simulink model "ctrl_HSMBObserver"  (R2015a)
settings: Solver=ode3  StartTime=0.0  StopTime=inf  FixedStep=0.01  RelTol=1e-3
values from neighbouring files (symbols this model uses):
  C = [C1;C2;C3;C4;C5;C6]    [initfile.m]    (also in thrustallocationQuadraticFixed.m)
  D = 3.0/100    (= 0.03)    [initfile.m]    (also in thrustallocationQuadraticFixed.m = 0.0411111111111)
  eps_c = 5    [initfile.m]
  epsilon = 0.5    [initfile.m]    (also in thrustallocationPseudo.m = u(10); thrustallocationQuadraticFixed.m = u(10))
  hd = c2d(H1,0.01,'foh')    [initfile.m]
  hd2 = c2d(H2,0.01,'zoh')    [initfile.m]
  I_s = 25000 /747225    (= 0.0334571246947)    [initfile.m]
  k_cc = 1    [initfile.m]
  K_omega = 0.3    [initfile.m]
  K_q1f = 0.0113    [initfile.m]
  K_q1r = K_q1f    (= 0.0113)    [initfile.m]
  K_q2f = 0.0117    [initfile.m]
  K_q2r = K_q2f    (= 0.0117)    [initfile.m]
  K_q3f = 0.0113    [initfile.m]
  K_q3r = K_q3f    (= 0.0113)    [initfile.m]
  K_q4f = 0.0169    [initfile.m]
  K_q4r = K_q4f    (= 0.0169)    [initfile.m]
  K_q5f = 0.0144    [initfile.m]
  K_q5r = K_q5f    (= 0.0144)    [initfile.m]
  K_q6f = 0.0168    [initfile.m]
  K_q6r = K_q6f    (= 0.0168)    [initfile.m]
  K_T1f = 0.3763    [initfile.m]
  K_T1r = K_T1f    (= 0.3763)    [initfile.m]
  K_T2f = 0.3901    [initfile.m]
  K_T2r = K_T2f    (= 0.3901)    [initfile.m]
  K_T3f = 0.3776    [initfile.m]
  K_T3r = K_T3f    (= 0.3776)    [initfile.m]
  K_T4f = 0.5641    [initfile.m]
  K_T4r = K_T4f    (= 0.5641)    [initfile.m]
  K_T5f = 0.4799    [initfile.m]
  K_T5r = K_T5f    (= 0.4799)    [initfile.m]
  K_T6f = 0.5588    [initfile.m]
  K_T6r = K_T6f    (= 0.5588)    [initfile.m]
  Kp = 3.3    [initfile.m]
  Max_Acceleration = 5    [initfile.m]
  Max_rotation = 12*sqrt(lambda)    [initfile.m]
  Max_thrust = 1.5    [initfile.m]
  Min_thrust = -0.8    [initfile.m]
  n_c = 5    [initfile.m]
  n_max = 152    [initfile.m]
  p_cc = 0.5    [initfile.m]
  pwm_thr1_backward = coeffvalues(ForceToPWM)    [initfile.m]
  pwm_thr1_forward = coeffvalues(ForceToPWM)    [initfile.m]
  pwm_thr2_backward = coeffvalues(ForceToPWM)    [initfile.m]
  pwm_thr2_forward = coeffvalues(ForceToPWM)    [initfile.m]
  pwm_thr3_backward = coeffvalues(ForceToPWM)    [initfile.m]
  pwm_thr3_forward = coeffvalues(ForceToPWM)    [initfile.m]
  pwm_thr4_backward = coeffvalues(ForceToPWM)    [initfile.m]
  pwm_thr4_forward = coeffvalues(ForceToPWM)    [initfile.m]
  pwm_thr5_backward = coeffvalues(ForceToPWM)    [initfile.m]
  pwm_thr5_forward = coeffvalues(ForceToPWM)    [initfile.m]
  pwm_thr6_backward = coeffvalues(ForceToPWM)    [initfile.m]
  pwm_thr6_forward = coeffvalues(ForceToPWM)    [initfile.m]
  Q_f0 = 0.3    [initfile.m]
  r_cc = 4    [initfile.m]
  Rho = Rho_m    (= 1000)    [initfile.m]
  ts = [-1 0]    [thrustallocationPseudo.m]    (also in thrustallocationQuadraticFixed.m)
undefined symbols (not defined in the file or in its folder): AFB, arm, Att, Control, Damping, FaultDet, Glob, Grip, IntActionType, Mass, NPO, Obs, Omg0_min, Q_max, ReferenceMdl, Sensor, Sim, SwLogic, tau, Thruster, Thruster_lock
libraries: dspmtrx3 x14, marine_gnc x11, simulink_extras x9, dspstat3 x9, simulink x9, dsparch4 x6, dspspect3 x6
(part 4 of 7)

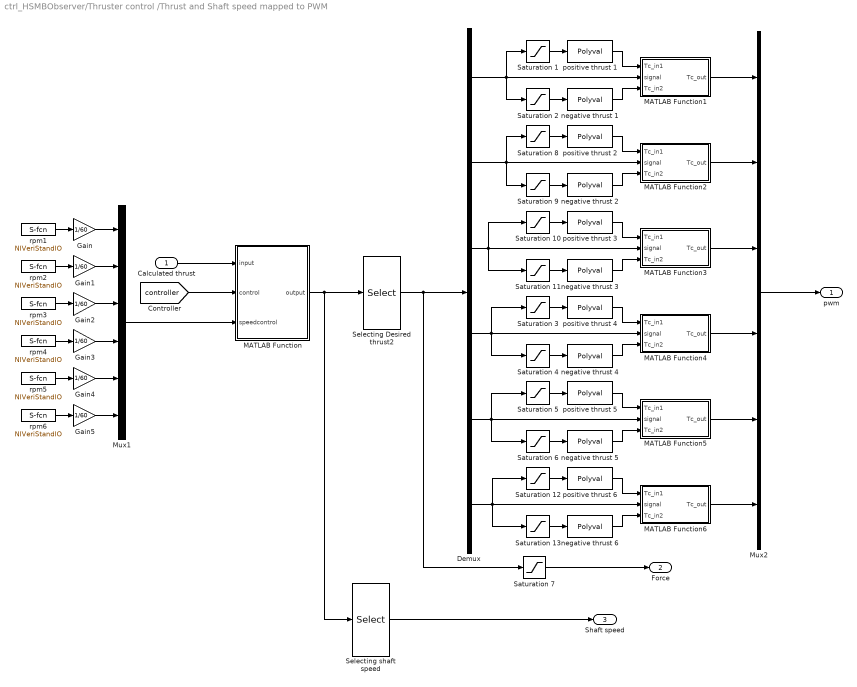
== system ctrl_HSMBObserver/Thruster control /Thrust and Shaft speed mapped to PWM ==
  Calculated thrust : Inport
  Demux : Demux  Outputs=6
  Gain{,1..5} (6 alike) : Gain  Gain=1/60
  MATLAB Function : MATLAB Function  TreatAsAtomicUnit=on
  MATLAB Function1 : MATLAB Function  TreatAsAtomicUnit=on
  MATLAB Function2 : MATLAB Function  TreatAsAtomicUnit=on
  MATLAB Function3 : MATLAB Function  TreatAsAtomicUnit=on
  MATLAB Function4 : MATLAB Function  TreatAsAtomicUnit=on
  MATLAB Function5 : MATLAB Function  TreatAsAtomicUnit=on
  MATLAB Function6 : MATLAB Function  TreatAsAtomicUnit=on
  Mux1 : Mux  Inputs=6
  Mux2 : Mux  Inputs=6
  Saturation {1,3,5,8,10,12} (6 alike) : Saturate  UpperLimit=Max_thrust  LowerLimit=0
  Saturation {2,4,6,9,11,13} (6 alike) : Saturate  UpperLimit=0  LowerLimit=Min_thrust
  Saturation 7 : Saturate  UpperLimit=Max_thrust  LowerLimit=-Max_thrust
  Selecting Desired thrust2 : Selector  InputPortWidth=12  Indices=[1 3 5 7 9 11]
  Selecting shaft speed : Selector  InputPortWidth=12  Indices=[2 4 6 8 10 12]
  negative thrust 1 : Polyval  Coefs=pwm_thr1_backward
  negative thrust 2 : Polyval  Coefs=pwm_thr2_backward
  negative thrust 3 : Polyval  Coefs=pwm_thr3_backward
  negative thrust 4 : Polyval  Coefs=pwm_thr4_backward
  negative thrust 5 : Polyval  Coefs=pwm_thr5_backward
  negative thrust 6 : Polyval  Coefs=pwm_thr6_backward
  positive thrust 1 : Polyval  Coefs=pwm_thr1_forward
  positive thrust 2 : Polyval  Coefs=pwm_thr2_forward
  positive thrust 3 : Polyval  Coefs=pwm_thr3_forward
  positive thrust 4 : Polyval  Coefs=pwm_thr4_forward
  positive thrust 5 : Polyval  Coefs=pwm_thr5_forward
  positive thrust 6 : Polyval  Coefs=pwm_thr6_forward
  "rpm1 " : S-Function  Priority=1  FunctionName=NIVeriStandIO  Parameters=width dtype portnum stime stype btype  mask(NI VeriStand Inport){portnum=1, width=-1, stime=-1, dtype=auto, stype=auto, btype=1}
      mask prompts: portnum "Port number:"; width "Port dimensions (-1 for dynamically sized):"; stime "Sample time (-1 for inherited):"; dtype "Data type:"; stype "Signal type:"; btype "Block type:"
      mask help: Use this inport on any level of nested subsystems to allow NI VeriStand software to map signals to it.
      mask init:
      | NIVeriStandIO_init;
      settings: CopyFcn=NIVeriStand_MDL_functions('', 'IO_copy');  DeleteFcn=NIVeriStand_MDL_functions('', 'IO_delete');  MoveFcn=set_param(gcb, 'Mask', 'on');
      mask Callback portnum: NIVeriStand_MDL_functions('', 'IO_setportnum');
      mask TypeOptions dtype: auto | double | single | int8 | uint8 | int16 | uint16 | int32 | uint32 | boolean
      mask Callback dtype: NIVeriStand_MDL_functions('', 'IO_booleansignal');
      mask TypeOptions stype: auto | real | complex
      mask Display:
      | patch([-x x], [-y y], [.90980 .81960 .32156]);
      | plot([xrad -x x xrad], [yrad -y y yrad]);
      | fprintf('NI In%d', portnum);
  rpm2 : S-Function  Priority=2  FunctionName=NIVeriStandIO  Parameters=width dtype portnum stime stype btype  mask(NI VeriStand Inport){portnum=2, width=-1, stime=-1, dtype=auto, stype=auto, btype=1}
      mask prompts: portnum "Port number:"; width "Port dimensions (-1 for dynamically sized):"; stime "Sample time (-1 for inherited):"; dtype "Data type:"; stype "Signal type:"; btype "Block type:"
      mask help: Use this inport on any level of nested subsystems to allow NI VeriStand software to map signals to it.
      mask init:
      | NIVeriStandIO_init;
      settings: CopyFcn=NIVeriStand_MDL_functions('', 'IO_copy');  DeleteFcn=NIVeriStand_MDL_functions('', 'IO_delete');  MoveFcn=set_param(gcb, 'Mask', 'on');
      mask Callback portnum: NIVeriStand_MDL_functions('', 'IO_setportnum');
      mask TypeOptions dtype: auto | double | single | int8 | uint8 | int16 | uint16 | int32 | uint32 | boolean
      mask Callback dtype: NIVeriStand_MDL_functions('', 'IO_booleansignal');
      mask TypeOptions stype: auto | real | complex
      mask Display:
      | patch([-x x], [-y y], [.90980 .81960 .32156]);
      | plot([xrad -x x xrad], [yrad -y y yrad]);
      | fprintf('NI In%d', portnum);
  rpm3 : S-Function  Priority=3  FunctionName=NIVeriStandIO  Parameters=width dtype portnum stime stype btype  mask(NI VeriStand Inport){portnum=3, width=-1, stime=-1, dtype=auto, stype=auto, btype=1}
      mask prompts: portnum "Port number:"; width "Port dimensions (-1 for dynamically sized):"; stime "Sample time (-1 for inherited):"; dtype "Data type:"; stype "Signal type:"; btype "Block type:"
      mask help: Use this inport on any level of nested subsystems to allow NI VeriStand software to map signals to it.
      mask init:
      | NIVeriStandIO_init;
      settings: CopyFcn=NIVeriStand_MDL_functions('', 'IO_copy');  DeleteFcn=NIVeriStand_MDL_functions('', 'IO_delete');  MoveFcn=set_param(gcb, 'Mask', 'on');
      mask Callback portnum: NIVeriStand_MDL_functions('', 'IO_setportnum');
      mask TypeOptions dtype: auto | double | single | int8 | uint8 | int16 | uint16 | int32 | uint32 | boolean
      mask Callback dtype: NIVeriStand_MDL_functions('', 'IO_booleansignal');
      mask TypeOptions stype: auto | real | complex
      mask Display:
      | patch([-x x], [-y y], [.90980 .81960 .32156]);
      | plot([xrad -x x xrad], [yrad -y y yrad]);
      | fprintf('NI In%d', portnum);
  rpm4 : S-Function  Priority=4  FunctionName=NIVeriStandIO  Parameters=width dtype portnum stime stype btype  mask(NI VeriStand Inport){portnum=4, width=-1, stime=-1, dtype=auto, stype=auto, btype=1}
      mask prompts: portnum "Port number:"; width "Port dimensions (-1 for dynamically sized):"; stime "Sample time (-1 for inherited):"; dtype "Data type:"; stype "Signal type:"; btype "Block type:"
      mask help: Use this inport on any level of nested subsystems to allow NI VeriStand software to map signals to it.
      mask init:
      | NIVeriStandIO_init;
      settings: CopyFcn=NIVeriStand_MDL_functions('', 'IO_copy');  DeleteFcn=NIVeriStand_MDL_functions('', 'IO_delete');  MoveFcn=set_param(gcb, 'Mask', 'on');
      mask Callback portnum: NIVeriStand_MDL_functions('', 'IO_setportnum');
      mask TypeOptions dtype: auto | double | single | int8 | uint8 | int16 | uint16 | int32 | uint32 | boolean
      mask Callback dtype: NIVeriStand_MDL_functions('', 'IO_booleansignal');
      mask TypeOptions stype: auto | real | complex
      mask Display:
      | patch([-x x], [-y y], [.90980 .81960 .32156]);
      | plot([xrad -x x xrad], [yrad -y y yrad]);
      | fprintf('NI In%d', portnum);
  rpm5 : S-Function  Priority=5  FunctionName=NIVeriStandIO  Parameters=width dtype portnum stime stype btype  mask(NI VeriStand Inport){portnum=5, width=-1, stime=-1, dtype=auto, stype=auto, btype=1}
      mask prompts: portnum "Port number:"; width "Port dimensions (-1 for dynamically sized):"; stime "Sample time (-1 for inherited):"; dtype "Data type:"; stype "Signal type:"; btype "Block type:"
      mask help: Use this inport on any level of nested subsystems to allow NI VeriStand software to map signals to it.
      mask init:
      | NIVeriStandIO_init;
      settings: CopyFcn=NIVeriStand_MDL_functions('', 'IO_copy');  DeleteFcn=NIVeriStand_MDL_functions('', 'IO_delete');  MoveFcn=set_param(gcb, 'Mask', 'on');
      mask Callback portnum: NIVeriStand_MDL_functions('', 'IO_setportnum');
      mask TypeOptions dtype: auto | double | single | int8 | uint8 | int16 | uint16 | int32 | uint32 | boolean
      mask Callback dtype: NIVeriStand_MDL_functions('', 'IO_booleansignal');
      mask TypeOptions stype: auto | real | complex
      mask Display:
      | patch([-x x], [-y y], [.90980 .81960 .32156]);
      | plot([xrad -x x xrad], [yrad -y y yrad]);
      | fprintf('NI In%d', portnum);
  rpm6 : S-Function  Priority=6  FunctionName=NIVeriStandIO  Parameters=width dtype portnum stime stype btype  mask(NI VeriStand Inport){portnum=6, width=-1, stime=-1, dtype=auto, stype=auto, btype=1}
      mask prompts: portnum "Port number:"; width "Port dimensions (-1 for dynamically sized):"; stime "Sample time (-1 for inherited):"; dtype "Data type:"; stype "Signal type:"; btype "Block type:"
      mask help: Use this inport on any level of nested subsystems to allow NI VeriStand software to map signals to it.
      mask init:
      | NIVeriStandIO_init;
      settings: CopyFcn=NIVeriStand_MDL_functions('', 'IO_copy');  DeleteFcn=NIVeriStand_MDL_functions('', 'IO_delete');  MoveFcn=set_param(gcb, 'Mask', 'on');
      mask Callback portnum: NIVeriStand_MDL_functions('', 'IO_setportnum');
      mask TypeOptions dtype: auto | double | single | int8 | uint8 | int16 | uint16 | int32 | uint32 | boolean
      mask Callback dtype: NIVeriStand_MDL_functions('', 'IO_booleansignal');
      mask TypeOptions stype: auto | real | complex
      mask Display:
      | patch([-x x], [-y y], [.90980 .81960 .32156]);
      | plot([xrad -x x xrad], [yrad -y y yrad]);
      | fprintf('NI In%d', portnum);
  pwm : Outport
  Force : Outport  Port=2
  "Shaft speed " : Outport  Port=3
  wires:
  MATLAB Function/1(output) -> Selecting shaft speed/1, Selecting Desired thrust2/1
  [controller] -> MATLAB Function/2(control)
  Mux2/1 -> pwm/1
  Selecting Desired thrust2/1 -> Saturation 7/1, Demux/1
  Selecting shaft speed/1 -> "Shaft speed "/1
  Saturation 7/1 -> Force/1
  "rpm1 "/1 -> Gain/1
  rpm2/1 -> Gain1/1
  rpm3/1 -> Gain2/1
  rpm4/1 -> Gain3/1
  rpm5/1 -> Gain4/1
  rpm6/1 -> Gain5/1
  Mux1/1 -> MATLAB Function/3(speedcontrol)
  positive thrust 1/1 -> MATLAB Function1/1(Tc_in1)
  negative thrust 1/1 -> MATLAB Function1/3(Tc_in2)
  Demux/1 -> Saturation 1/1, MATLAB Function1/2(signal), Saturation 2/1
  MATLAB Function1/1(Tc_out) -> Mux2/1
  Saturation 1/1 -> positive thrust 1/1
  Saturation 2/1 -> negative thrust 1/1
  positive thrust 2/1 -> MATLAB Function2/1(Tc_in1)
  negative thrust 2/1 -> MATLAB Function2/3(Tc_in2)
  Demux/2 -> Saturation 9/1, Saturation 8/1, MATLAB Function2/2(signal)
  MATLAB Function2/1(Tc_out) -> Mux2/2
  Saturation 8/1 -> positive thrust 2/1
  Saturation 9/1 -> negative thrust 2/1
  positive thrust 3/1 -> MATLAB Function3/1(Tc_in1)
  negative thrust 3/1 -> MATLAB Function3/3(Tc_in2)
  Demux/3 -> Saturation 11/1, MATLAB Function3/2(signal), Saturation 10/1
  MATLAB Function3/1(Tc_out) -> Mux2/3
  Saturation 10/1 -> positive thrust 3/1
  Saturation 11/1 -> negative thrust 3/1
  positive thrust 4/1 -> MATLAB Function4/1(Tc_in1)
  negative thrust 4/1 -> MATLAB Function4/3(Tc_in2)
  MATLAB Function4/1(Tc_out) -> Mux2/4
  Saturation 3/1 -> positive thrust 4/1
  Saturation 4/1 -> negative thrust 4/1
  Demux/4 -> Saturation 3/1, Saturation 4/1, MATLAB Function4/2(signal)
  positive thrust 5/1 -> MATLAB Function5/1(Tc_in1)
  negative thrust 5/1 -> MATLAB Function5/3(Tc_in2)
  MATLAB Function5/1(Tc_out) -> Mux2/5
  Saturation 5/1 -> positive thrust 5/1
  Saturation 6/1 -> negative thrust 5/1
  Demux/5 -> Saturation 5/1, MATLAB Function5/2(signal), Saturation 6/1
  positive thrust 6/1 -> MATLAB Function6/1(Tc_in1)
  negative thrust 6/1 -> MATLAB Function6/3(Tc_in2)
  MATLAB Function6/1(Tc_out) -> Mux2/6
  Saturation 12/1 -> positive thrust 6/1
  Saturation 13/1 -> negative thrust 6/1
  Demux/6 -> Saturation 13/1, Saturation 12/1, MATLAB Function6/2(signal)
  Gain/1 -> Mux1/1
  Gain5/1 -> Mux1/6
  Gain4/1 -> Mux1/5
  Gain3/1 -> Mux1/4
  Gain2/1 -> Mux1/3
  Gain1/1 -> Mux1/2
  Calculated thrust/1 -> MATLAB Function/1(input)

== system ctrl_HSMBObserver/Thruster control /Thruster 1 ==
  Desired thrust 1 : Inport
  shaft speed : Inport  Port=2
  Constant : Constant  Value=hd2.den{1,1}
  Constant1 : Constant  Value=hd2.num{1,1}
  Delay : Delay  DelayLength=1  InitialCondition=0
  Discrete Transfer Fcn : DiscreteTransferFcn  NumeratorSource=Input port  DenominatorSource=Input port  Denominator=[0.2 1]  SampleTime=0.01  a0EqualsOne=on
      settings: InputPortMap=u0,p1,p3
  Losses (placeholder) : Constant  Value=0
  Propeller Hydrodynamics : Subsystem
  Shaft dynamics : Subsystem
  Thruster control : Subsystem
  "Commanded thrust " : Outport
  Shaft speed : Outport  Port=2
  wires:
  Losses (placeholder)/1 -> Propeller Hydrodynamics/1(env)
  Shaft dynamics/1(n) -> Shaft speed/1, Propeller Hydrodynamics/2(n)
  Propeller Hydrodynamics/2(Qa) -> Delay/1
  Propeller Hydrodynamics/1(Ta) -> "Commanded thrust "/1
  Thruster control/1(Qc) -> Discrete Transfer Fcn/1
  Constant1/1 -> Discrete Transfer Fcn/2
  Constant/1 -> Discrete Transfer Fcn/3
  Discrete Transfer Fcn/1 -> Shaft dynamics/1(Qm)
  shaft speed/1 -> Thruster control/2(n)
  Delay/1 -> Shaft dynamics/2(Qa)
  Desired thrust 1/1 -> Thruster control/1("T_d ")

== system ctrl_HSMBObserver/Thruster control /Thruster 2 ==
  Desired thrust 1 : Inport
  shaft speed : Inport  Port=2
  Constant : Constant  Value=hd2.den{1,1}
  Constant1 : Constant  Value=hd2.num{1,1}
  Delay : Delay  DelayLength=1  InitialCondition=0
  Discrete Transfer Fcn : DiscreteTransferFcn  NumeratorSource=Input port  DenominatorSource=Input port  Denominator=[0.2 1]  SampleTime=0.01  a0EqualsOne=on
      settings: InputPortMap=u0,p1,p3
  Losses (placeholder) : Constant  Value=0
  Propeller Hydrodynamics : Subsystem
  Shaft dynamics : Subsystem
  Thruster control : Subsystem
  "Commanded thrust " : Outport
  Shaft speed : Outport  Port=2
  wires:
  Losses (placeholder)/1 -> Propeller Hydrodynamics/1(env)
  Shaft dynamics/1(n) -> Propeller Hydrodynamics/2(n), Shaft speed/1
  Propeller Hydrodynamics/2(Qa) -> Delay/1
  Thruster control/1(Qc) -> Discrete Transfer Fcn/1
  Discrete Transfer Fcn/1 -> Shaft dynamics/1(Qm)
  Desired thrust 1/1 -> Thruster control/1("T_d ")
  Propeller Hydrodynamics/1(Ta) -> "Commanded thrust "/1
  Constant1/1 -> Discrete Transfer Fcn/2
  Constant/1 -> Discrete Transfer Fcn/3
  shaft speed/1 -> Thruster control/2(n)
  Delay/1 -> Shaft dynamics/2(Qa)

== system ctrl_HSMBObserver/Thruster control /Thruster 3 ==
  Desired thrust 1 : Inport
  shaft speed : Inport  Port=2
  Constant : Constant  Value=hd2.den{1,1}
  Constant1 : Constant  Value=hd2.num{1,1}
  Delay : Delay  DelayLength=1  InitialCondition=0
  Discrete Transfer Fcn : DiscreteTransferFcn  NumeratorSource=Input port  DenominatorSource=Input port  Denominator=[0.2 1]  SampleTime=0.01  a0EqualsOne=on
      settings: InputPortMap=u0,p1,p3
  Losses (placeholder) : Constant  Value=0
  Propeller Hydrodynamics : Subsystem
  Shaft dynamics : Subsystem
  Thruster control : Subsystem
  "Commanded thrust " : Outport
  Shaft speed : Outport  Port=2
  wires:
  Losses (placeholder)/1 -> Propeller Hydrodynamics/1(env)
  Shaft dynamics/1(n) -> Propeller Hydrodynamics/2(n), Shaft speed/1
  Propeller Hydrodynamics/2(Qa) -> Delay/1
  Thruster control/1(Qc) -> Discrete Transfer Fcn/1
  Discrete Transfer Fcn/1 -> Shaft dynamics/1(Qm)
  Desired thrust 1/1 -> Thruster control/1("T_d ")
  Propeller Hydrodynamics/1(Ta) -> "Commanded thrust "/1
  Constant1/1 -> Discrete Transfer Fcn/2
  Constant/1 -> Discrete Transfer Fcn/3
  shaft speed/1 -> Thruster control/2(n)
  Delay/1 -> Shaft dynamics/2(Qa)

== system ctrl_HSMBObserver/Thruster control /Thruster 4 ==
  Desired thrust 1 : Inport
  shaft speed : Inport  Port=2
  Constant : Constant  Value=hd2.den{1,1}
  Constant1 : Constant  Value=hd2.num{1,1}
  Delay : Delay  DelayLength=1  InitialCondition=0
  Discrete Transfer Fcn : DiscreteTransferFcn  NumeratorSource=Input port  DenominatorSource=Input port  Denominator=[0.2 1]  SampleTime=0.01  a0EqualsOne=on
      settings: InputPortMap=u0,p1,p3
  Losses (placeholder) : Constant  Value=0
  Propeller Hydrodynamics : Subsystem
  Shaft dynamics : Subsystem
  Thruster control : Subsystem
  "Commanded thrust " : Outport
  Shaft speed : Outport  Port=2
  wires:
  Losses (placeholder)/1 -> Propeller Hydrodynamics/1(env)
  Shaft dynamics/1(n) -> Propeller Hydrodynamics/2(n), Shaft speed/1
  Propeller Hydrodynamics/2(Qa) -> Delay/1
  Thruster control/1(Qc) -> Discrete Transfer Fcn/1
  Discrete Transfer Fcn/1 -> Shaft dynamics/1(Qm)
  Desired thrust 1/1 -> Thruster control/1("T_d ")
  Propeller Hydrodynamics/1(Ta) -> "Commanded thrust "/1
  Constant1/1 -> Discrete Transfer Fcn/2
  Constant/1 -> Discrete Transfer Fcn/3
  shaft speed/1 -> Thruster control/2(n)
  Delay/1 -> Shaft dynamics/2(Qa)

== system ctrl_HSMBObserver/Thruster control /Thruster 5 ==
  Desired thrust 1 : Inport
  shaft speed : Inport  Port=2
  Constant : Constant  Value=hd2.den{1,1}
  Constant1 : Constant  Value=hd2.num{1,1}
  Delay : Delay  DelayLength=1  InitialCondition=0
  Discrete Transfer Fcn : DiscreteTransferFcn  NumeratorSource=Input port  DenominatorSource=Input port  Denominator=[0.2 1]  SampleTime=0.01  a0EqualsOne=on
      settings: InputPortMap=u0,p1,p3
  Losses (placeholder) : Constant  Value=0
  Propeller Hydrodynamics : Subsystem
  Shaft dynamics : Subsystem
  Thruster control : Subsystem
  "Commanded thrust " : Outport
  Shaft speed : Outport  Port=2
  wires:
  Losses (placeholder)/1 -> Propeller Hydrodynamics/1(env)
  Shaft dynamics/1(n) -> Propeller Hydrodynamics/2(n), Shaft speed/1
  Propeller Hydrodynamics/2(Qa) -> Delay/1
  Thruster control/1(Qc) -> Discrete Transfer Fcn/1
  Discrete Transfer Fcn/1 -> Shaft dynamics/1(Qm)
  Desired thrust 1/1 -> Thruster control/1("T_d ")
  Propeller Hydrodynamics/1(Ta) -> "Commanded thrust "/1
  Constant1/1 -> Discrete Transfer Fcn/2
  Constant/1 -> Discrete Transfer Fcn/3
  shaft speed/1 -> Thruster control/2(n)
  Delay/1 -> Shaft dynamics/2(Qa)

== system ctrl_HSMBObserver/Thruster control /Thruster 6 ==
  Desired thrust 1 : Inport
  shaft speed : Inport  Port=2
  Constant : Constant  Value=hd2.den{1,1}
  Constant1 : Constant  Value=hd2.num{1,1}
  Delay : Delay  DelayLength=1  InitialCondition=0
  Discrete Transfer Fcn : DiscreteTransferFcn  NumeratorSource=Input port  DenominatorSource=Input port  Denominator=[0.2 1]  SampleTime=0.01  a0EqualsOne=on
      settings: InputPortMap=u0,p1,p3
  Losses (placeholder) : Constant  Value=0
  Propeller Hydrodynamics : Subsystem
  Shaft dynamics : Subsystem
  Thruster control : Subsystem
  "Commanded thrust " : Outport
  Shaft speed : Outport  Port=2
  wires:
  Losses (placeholder)/1 -> Propeller Hydrodynamics/1(env)
  Shaft dynamics/1(n) -> Propeller Hydrodynamics/2(n), Shaft speed/1
  Propeller Hydrodynamics/2(Qa) -> Delay/1
  Thruster control/1(Qc) -> Discrete Transfer Fcn/1
  Discrete Transfer Fcn/1 -> Shaft dynamics/1(Qm)
  Desired thrust 1/1 -> Thruster control/1("T_d ")
  Propeller Hydrodynamics/1(Ta) -> "Commanded thrust "/1
  Constant1/1 -> Discrete Transfer Fcn/2
  Constant/1 -> Discrete Transfer Fcn/3
  shaft speed/1 -> Thruster control/2(n)
  Delay/1 -> Shaft dynamics/2(Qa)

== system ctrl_HSMBObserver/To meters and radians, noise and sampling/SampleTime ==
  Rate : Inport
  5 Hz GPS : ZeroOrderHold  SampleTime=Sensor.GPS.SampleTime
  5 Hz GPS1 : ZeroOrderHold  SampleTime=Sensor.GPS.SampleTime
  50 Hz compass2 : ZeroOrderHold  SampleTime=Sensor.Compass.SampleTime
  Demux : Demux  Outputs=3
  Mux : Mux  Inputs=3
  Rate Transition1 : RateTransition  Deterministic=off
  Rate Transition2 : RateTransition  Deterministic=off
  Rate Transition3 : RateTransition  Deterministic=off
  Scope : Scope
      settings: YMin=-7.75  YMax=-2.25  SaveName=ScopeData199
  ReducedRates : Outport
  wires:
  Rate/1 -> Demux/1
  Demux/1 -> 5 Hz GPS/1
  5 Hz GPS/1 -> Rate Transition2/1
  Demux/2 -> 5 Hz GPS1/1
  5 Hz GPS1/1 -> Rate Transition1/1
  Demux/3 -> 50 Hz compass2/1
  50 Hz compass2/1 -> Rate Transition3/1
  Mux/1 -> ReducedRates/1
  Rate Transition2/1 -> Scope/1, Mux/1
  Rate Transition1/1 -> Mux/2
  Rate Transition3/1 -> Mux/3

== system ctrl_HSMBObserver/To meters and radians, noise and sampling/Sensor noise models ==
  note: Compass: yaw
  note: GPS: surge, sway
  Compass measurement noise module : Subsystem
  Mux : Mux  Inputs=2
  Position (x,y) GPS measurement noise module : Subsystem
  Eta_noise : Outport
  wires:
  Mux/1 -> Eta_noise/1
  Compass measurement noise module/1(Psi_noised) -> Mux/2
  Position (x,y) GPS measurement noise module/1(noised_pos (x.y)) -> Mux/1

== system ctrl_HSMBObserver/To meters and radians, noise and sampling/[-inf inf] to [-pi pi]1 ==
  note: x
  note: r
  x [-inf inf] : Inport
  Constant : Constant  Value=2*pi
  Gain : Gain  Gain=pi  SaturateOnIntegerOverflow=on  OutDataTypeStr=Inherit: Same as input  ParamDataTypeStr=Inherit: Same as input
  Math Function : Math  Operator=rem  SaturateOnIntegerOverflow=on
  Saturation : Saturate  UpperLimit=1e10  LowerLimit=-1e10
  Sign : Signum
  Sum : Sum  Inputs=|+-  SaturateOnIntegerOverflow=on
  Sum1 : Sum  Inputs=|++  SaturateOnIntegerOverflow=on
  y [-pi pi] : Outport
  wires:
  x [-inf inf]/1 -> Saturation/1
  Sign/1 -> Gain/1
  Gain/1 -> Sum/2, Sum1/2
  Sum1/1 -> Math Function/1
  Constant/1 -> Math Function/2
  Math Function/1 -> Sum/1
  Sum/1 -> y [-pi pi]/1
  Saturation/1 -> Sum1/1, Sign/1

== system ctrl_HSMBObserver/To meters and radians, noise and sampling/[-inf inf] to [-pi pi]2 ==
  note: x
  note: r
  x [-inf inf] : Inport
  Constant : Constant  Value=2*pi
  Gain : Gain  Gain=pi  SaturateOnIntegerOverflow=on  OutDataTypeStr=Inherit: Same as input  ParamDataTypeStr=Inherit: Same as input
  Math Function : Math  Operator=rem  SaturateOnIntegerOverflow=on
  Saturation : Saturate  UpperLimit=1e10  LowerLimit=-1e10
  Sign : Signum
  Sum : Sum  Inputs=|+-  SaturateOnIntegerOverflow=on
  Sum1 : Sum  Inputs=|++  SaturateOnIntegerOverflow=on
  y [-pi pi] : Outport
  wires:
  x [-inf inf]/1 -> Saturation/1
  Sign/1 -> Gain/1
  Gain/1 -> Sum/2, Sum1/2
  Sum1/1 -> Math Function/1
  Constant/1 -> Math Function/2
  Math Function/1 -> Sum/1
  Sum/1 -> y [-pi pi]/1
  Saturation/1 -> Sum1/1, Sign/1

== system ctrl_HSMBObserver/To meters and radians, noise and sampling/[-inf inf] to [-pi pi]3 ==
  note: x
  note: r
  x [-inf inf] : Inport
  Constant : Constant  Value=2*pi
  Gain : Gain  Gain=pi  SaturateOnIntegerOverflow=on  OutDataTypeStr=Inherit: Same as input  ParamDataTypeStr=Inherit: Same as input
  Math Function : Math  Operator=rem  SaturateOnIntegerOverflow=on
  Saturation : Saturate  UpperLimit=1e10  LowerLimit=-1e10
  Sign : Signum
  Sum : Sum  Inputs=|+-  SaturateOnIntegerOverflow=on
  Sum1 : Sum  Inputs=|++  SaturateOnIntegerOverflow=on
  y [-pi pi] : Outport
  wires:
  x [-inf inf]/1 -> Saturation/1
  Sign/1 -> Gain/1
  Gain/1 -> Sum/2, Sum1/2
  Sum1/1 -> Math Function/1
  Constant/1 -> Math Function/2
  Math Function/1 -> Sum/1
  Sum/1 -> y [-pi pi]/1
  Saturation/1 -> Sum1/1, Sign/1

== system ctrl_HSMBObserver/Hybrid Controller/Controllers/Subsystem ==
  acc_est : Inport
  acc_des : Inport  Port=2
  Enable : EnablePort
  Control3 : Scope  NumInputPorts=2
      settings: YMin=-4e+07~-7e+07  YMax=5.5e+07~8e+07  SaveName=ScopeData192
  Demux4 : Demux  Outputs=2
  Gain : Gain  Gain=-Control.Vessel.Ka  Multiplication=Matrix(K*u)  SaturateOnIntegerOverflow=on  OutDataTypeStr=Inherit: Same as input  ParamDataTypeStr=Inherit: Same as input
  Gain1 : Gain  Gain=1/AFB.TC
  Integrator : Integrator
  Selector : Selector  InputPortWidth=3  Indices=[1 2]
  Selector1 : Selector  InputPortWidth=3  Indices=[1 2]
  Sum : Sum  Inputs=|+-
  Sum3 : Sum  Inputs=+|-  SaturateOnIntegerOverflow=on
  Out1 : Outport
  wires:
  Selector1/1 -> Sum3/2
  acc_des/1 -> Selector1/1
  Sum3/1 -> Gain/1
  Selector/1 -> Sum3/1
  acc_est/1 -> Selector/1
  Gain/1 -> Sum/1, Demux4/1
  Demux4/1 -> Control3/1
  Demux4/2 -> Control3/2
  Sum/1 -> Gain1/1
  Integrator/1 -> Sum/2, Out1/1
  Gain1/1 -> Integrator/1

== system ctrl_HSMBObserver/Hybrid Controller/Controllers/Subsystem1 ==
  tau_timer : Inport
  u_PD_in : Inport  Port=2
  Constant : Constant  Value=tau.T_star
  Constant1 : Constant
  Constant2 : Constant
  Divide : Product  Inputs=*/
  If : If  IfExpression=u1 == 0  ShowElse=off
  Memory : Memory
  MinMax : MinMax  Inputs=2
  Product : Product
  Product1 : Product
  Scope{,1..5} (6 alike) : Scope
      Scope settings: YMin=20  YMax=20  SaveName=ScopeData157
      Scope1 settings: YMin=-2.25e+06  YMax=750000  SaveName=ScopeData158
      Scope2 settings: SaveName=ScopeData159
      Scope3 settings: YMin=-750000  YMax=2e+06  SaveName=ScopeData160
      Scope4 settings: YMin=-1.25e+06  YMax=3.25e+06  SaveName=ScopeData161
      Scope5 settings: YMin=-700000  YMax=500000  SaveName=ScopeData162
  Sum : Sum
  Sum1 : Sum  Inputs=+-|
  "fault, update to q == 1" : Subsystem  TreatAsAtomicUnit=on
  u_PD : Outport
  wires:
  [tau_timer] -> If/1
  [u_PD] -> Scope5/1, Product/2
  "fault, update to q == 1"/1(u_PD_hold) -> [u_PD_hold]
  [u_PD_hold] -> Scope1/1, Product1/2
  Product/1 -> Scope3/1, Sum/1
  Constant1/1 -> Sum1/1
  Product1/1 -> Scope2/1, Sum/2
  Sum1/1 -> Product1/1
  If/1 -> "fault, update to q == 1"/Action
  Sum/1 -> Scope4/1, u_PD/1
  Constant/1 -> Divide/2
  [tau_timer] -> Divide/1
  [lambda] -> Product/1
  [u_PD_hold_in] -> "fault, update to q == 1"/1(u_PD)
  [lambda] -> Sum1/2
  tau_timer/1 -> [tau_timer]
  u_PD_in/1 -> [u_PD]
  [u_PD] -> Memory/1
  Memory/1 -> [u_PD_hold_in]
  Constant2/1 -> MinMax/1
  Divide/1 -> MinMax/2
  MinMax/1 -> Scope/1, [lambda]

== system ctrl_HSMBObserver/Hybrid Controller/Controllers/Tau PD-control ==
  note: PD-control term in controller
      | Martin Austad, 2003
  Nu_des : Inport
  Eta_des : Inport  Port=2
  Eta_est : Inport  Port=3
  Nu_est : Inport  Port=4
  "Kp " : Inport  Port=5
  Kd : Inport  Port=6
  Scalefactor : Inport  Port=7
  Enable : EnablePort
  Clock : Clock
  Clock1 : Clock
  Constant : Constant
  Create Diagonal Matrix : dspmtrx3/Create Diagonal Matrix
  Create Diagonal Matrix1 : dspmtrx3/Create Diagonal Matrix
  "GNC: \"Transposed rotation matrix yaw: RTz_psi\"" : Subsystem
  Ki eta_tilde : MATLAB Function  TreatAsAtomicUnit=on
  Ki eta_tilde1 : MATLAB Function  TreatAsAtomicUnit=on
  MATLAB Function : MATLAB Function  TreatAsAtomicUnit=on
  MATLAB Function1 : MATLAB Function  TreatAsAtomicUnit=on
  Selector2 : Selector  InputPortWidth=3  Indices=[3]
  Sum : Sum  Inputs=+-|  SaturateOnIntegerOverflow=on
  Sum1 : Sum  Inputs=+-|  SaturateOnIntegerOverflow=on
  Sum2 : Sum  Inputs=|++
  tau_p : Outport
  tau_d : Outport  Port=2
  wires:
  Eta_est/1 -> Sum/1, Selector2/1
  Nu_est/1 -> Sum1/1
  Sum1/1 -> Ki eta_tilde1/1(nu_tilde)
  Nu_des/1 -> Sum1/2
  Eta_des/1 -> Sum/2
  Sum/1 -> "GNC: \"Transposed rotation matrix yaw: RTz_psi\""/2(eta_tilde)
  Selector2/1 -> "GNC: \"Transposed rotation matrix yaw: RTz_psi\""/1(psi)
  "GNC: \"Transposed rotation matrix yaw: RTz_psi\""/1(R_T*eta_tilde) -> Ki eta_tilde/1(eta_tilde_body)
  Ki eta_tilde1/1(tau_d) -> tau_d/1
  Ki eta_tilde/1(tau_p) -> tau_p/1
  "Kp "/1 -> Create Diagonal Matrix1/1
  MATLAB Function/1(Kp) -> Ki eta_tilde/2(Kp)
  Clock/1 -> MATLAB Function/2(t)
  Clock1/1 -> MATLAB Function1/2(t)
  MATLAB Function1/1(Kd) -> Ki eta_tilde1/2(Kd)
  [sf] -> MATLAB Function/3(sf)
  [sf] -> MATLAB Function1/3(sf)
  Kd/1 -> Create Diagonal Matrix/1
  Create Diagonal Matrix/1 -> MATLAB Function1/1(Kdin)
  Create Diagonal Matrix1/1 -> MATLAB Function/1(Kpin)
  Constant/1 -> Sum2/1
  Scalefactor/1 -> Sum2/2
  Sum2/1 -> [sf]

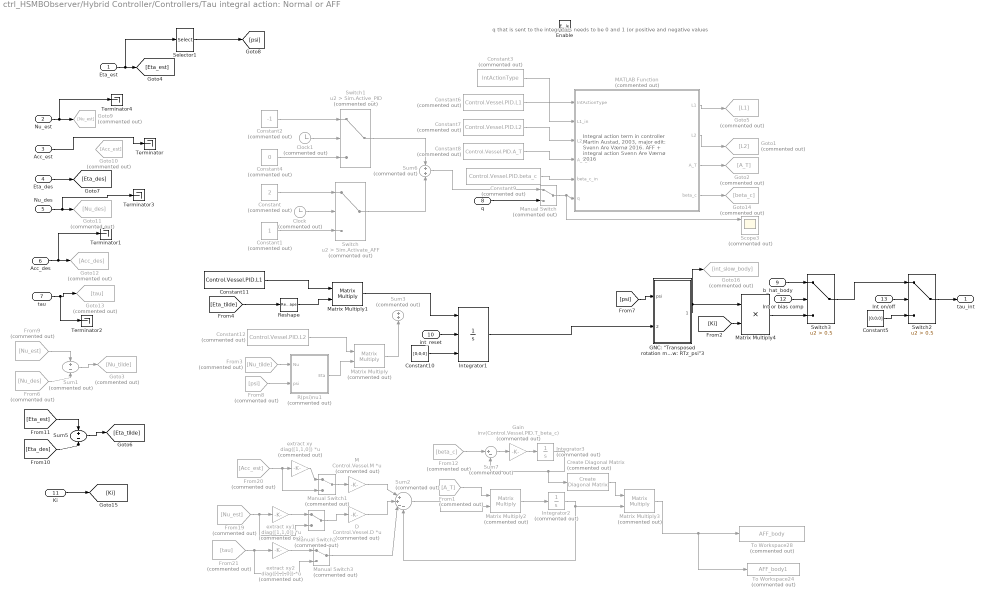
== system ctrl_HSMBObserver/Hybrid Controller/Controllers/Tau integral action: Normal or AFF ==
  note: q that is sent to the integrators needs to be 0 and 1 (or positive and negative values
  note: Integral action term in controller
      | Martin Austad, 2003,
      | major edit:
      | Svenn Are Værnø 2016.
      |
      | AFF + integral action
      | Svenn Are Værnø 2016
  Eta_est : Inport
  Nu_est : Inport  Port=2
  Acc_est : Inport  Port=3
  Eta_des : Inport  Port=4
  Nu_des : Inport  Port=5
  Acc_des : Inport  Port=6
  tau : Inport  Port=7
  q : Inport  Port=8
  b_hat_body : Inport  Port=9
  int_reset : Inport  Port=10
  Ki : Inport  Port=11
  Int or bias comp : Inport  Port=12
  Int on/off : Inport  Port=13
  Enable : EnablePort
  Clock : Clock  Commented=on
  Clock1 : Clock  Commented=on
  Constant : Constant  Commented=on  Value=2
  Constant1 : Constant  Commented=on
  Constant10 : Constant  Value=[0;0;0]
  Constant11 : Constant  Value=Control.Vessel.PID.L1
  Constant12 : Constant  Commented=on  Value=Control.Vessel.PID.L2
  Constant2 : Constant  Commented=on  Value=-1
  Constant3 : Constant  Commented=on  Value=IntActionType
  Constant4 : Constant  Commented=on  Value=0
  Constant5 : Constant  Value=[0;0;0]
  Constant6 : Constant  Commented=on  Value=Control.Vessel.PID.L1
  Constant7 : Constant  Commented=on  Value=Control.Vessel.PID.L2
  Constant8 : Constant  Commented=on  Value=Control.Vessel.PID.A_T
  Constant9 : Constant  Commented=on  Value=Control.Vessel.PID.beta_c
  Create Diagonal Matrix : dspmtrx3/Create Diagonal Matrix  Commented=on
  D : Gain  Commented=on  Gain=Control.Vessel.D  Multiplication=Matrix(K*u)
  From1 : From  Commented=on  GotoTag=A_T
  From12 : From  Commented=on  GotoTag=beta_c
  From19 : From  Commented=on  GotoTag=Nu_est
  From20 : From  Commented=on  GotoTag=Acc_est
  From21 : From  Commented=on  GotoTag=tau
  From3 : From  Commented=on  GotoTag=Nu_tilde
  From6 : From  Commented=on  GotoTag=Nu_des
  From8 : From  Commented=on  GotoTag=psi
  From9 : From  Commented=on  GotoTag=Nu_est
  "GNC: \"Transposed rotation matrix yaw: RTz_psi\"3" : Subsystem
  Gain : Gain  Commented=on  Gain=inv(Control.Vessel.PID.T_beta_c)
  Goto1 : Goto  Commented=on  GotoTag=L2
  Goto10 : Goto  Commented=on  GotoTag=Acc_est
  Goto11 : Goto  Commented=on  GotoTag=Nu_des
  Goto12 : Goto  Commented=on  GotoTag=Acc_des
  Goto13 : Goto  Commented=on  GotoTag=tau
  Goto14 : Goto  Commented=on  GotoTag=beta_c
  Goto16 : Goto  Commented=on  GotoTag=int_slow_body
  Goto2 : Goto  Commented=on  GotoTag=A_T
  Goto3 : Goto  Commented=on  GotoTag=Nu_tilde
  Goto5 : Goto  Commented=on  GotoTag=L1
  Goto9 : Goto  Commented=on  GotoTag=Nu_est
  Integrator1 : Integrator  ExternalReset=either  InitialConditionSource=external
  Integrator2 : Integrator  Commented=on  InitialCondition=[0;0;0]
  Integrator3 : Integrator  Commented=on  InitialCondition=[0;0;0]
  M : Gain  Commented=on  Gain=Control.Vessel.M  Multiplication=Matrix(K*u)
  MATLAB Function : MATLAB Function  Commented=on  TreatAsAtomicUnit=on
  Manual Switch{,1..3} (4 alike) : ManualSwitch  Commented=on
  Matrix Multiply : Product  Commented=on  Multiplication=Matrix(*)
  Matrix Multiply1 : Product  Multiplication=Matrix(*)
  Matrix Multiply2 : Product  Commented=on  Multiplication=Matrix(*)
  Matrix Multiply3 : Product  Commented=on  Multiplication=Matrix(*)
  Matrix Multiply4 : Product
  R(psi)nu1 : Subsystem  Commented=on
  Reshape : Reshape
  Scope3 : Scope  Commented=on  NumInputPorts=3
      settings: YMin=0.95~-1~-1  YMax=1.05~1~1  SaveName=ScopeData70
  Selector1 : Selector  InputPortWidth=3  Indices=[3]
  Sum1 : Sum  Commented=on  Inputs=+-  SaturateOnIntegerOverflow=on
  Sum2 : Sum  Commented=on  Inputs=|++--  SaturateOnIntegerOverflow=on
  Sum3 : Sum  Commented=on
  Sum5 : Sum  Inputs=+-  SaturateOnIntegerOverflow=on
  Sum6 : Sum  Commented=on
  Sum7 : Sum  Commented=on  Inputs=|+-  SaturateOnIntegerOverflow=on
  Switch : Switch  Commented=on  Criteria=u2 > Threshold  Threshold=Sim.Activate_AFF
  Switch1 : Switch  Commented=on  Criteria=u2 > Threshold  Threshold=Sim.Active_PID
  Switch2 : Switch  Criteria=u2 > Threshold  Threshold=0.5
  Switch3 : Switch  Criteria=u2 > Threshold  Threshold=0.5
  Terminator{,1..4} (5 alike) : Terminator
  To Workspace24 : ToWorkspace  Commented=on  VariableName=AFF_body1  SaveFormat=Timeseries  SampleTime=ts
  To Workspace28 : ToWorkspace  Commented=on  VariableName=AFF_body  SampleTime=ts
  extract xy : Gain  Commented=on  Gain=diag([1,1,0])  Multiplication=Matrix(K*u)
  extract xy1 : Gain  Commented=on  Gain=diag([1,1,0])  Multiplication=Matrix(K*u)
  extract xy2 : Gain  Commented=on  Gain=diag([1,1,0])  Multiplication=Matrix(K*u)
  tau_int : Outport  InitialOutput=[0,0,0]
  wires:
  M/1 -> Sum2/1
  D/1 -> Sum2/2
  MATLAB Function/2(L2) -> Goto1/1
  MATLAB Function/3(A_T) -> Goto2/1
  From19/1 -> Manual Switch2/2, extract xy1/1
  Constant1/1 -> Switch/3
  Clock/1 -> Switch/2
  Constant/1 -> Switch/1
  Constant4/1 -> Switch1/3
  Clock1/1 -> Switch1/2
  Constant2/1 -> Switch1/1
  Switch1/1 -> Sum6/1
  Switch/1 -> Sum6/2
  Manual Switch/1 -> Scope3/1, MATLAB Function/6(q)
  Eta_est/1 -> Selector1/1, [Eta_est]
  Nu_est/1 -> Terminator4/1, Goto9/1
  Eta_des/1 -> [Eta_des]
  Nu_des/1 -> Terminator3/1, Goto11/1
  Acc_des/1 -> Terminator1/1, Goto12/1
  From3/1 -> R(psi)nu1/1(Nu)
  From8/1 -> R(psi)nu1/2(psi)
  R(psi)nu1/1(Eta) -> Matrix Multiply/2
  Constant11/1 -> Matrix Multiply1/1
  [Eta_tilde] -> Reshape/1
  Sum6/1 -> Manual Switch/1
  q/1 -> Manual Switch/2
  Constant3/1 -> MATLAB Function/1(IntActionType)
  Constant6/1 -> MATLAB Function/2(L1_in)
  Constant7/1 -> MATLAB Function/3(L2_in)
  Constant8/1 -> MATLAB Function/4(A_T_in)
  MATLAB Function/1(L1) -> Goto5/1
  Matrix Multiply1/1 -> Integrator1/1
  Matrix Multiply/1 -> Sum3/2
  Selector1/1 -> [psi]
  From9/1 -> Sum1/1
  From6/1 -> Sum1/2
  Sum1/1 -> Goto3/1
  [Eta_est] -> Sum5/1
  [Eta_des] -> Sum5/2
  Sum5/1 -> [Eta_tilde]
  [psi] -> "GNC: \"Transposed rotation matrix yaw: RTz_psi\"3"/1(psi)
  Integrator1/1 -> "GNC: \"Transposed rotation matrix yaw: RTz_psi\"3"/2(int_NED)
  Sum2/1 -> Matrix Multiply2/2
  From1/1 -> Matrix Multiply2/1
  Matrix Multiply2/1 -> Integrator2/1
  Constant9/1 -> MATLAB Function/5(beta_c_in)
  MATLAB Function/4(beta_c) -> Goto14/1
  Integrator2/1 -> Matrix Multiply3/2, Sum2/4
  Matrix Multiply3/1 -> To Workspace24/1, To Workspace28/1
  From12/1 -> Sum7/1
  Sum7/1 -> Gain/1
  Gain/1 -> Integrator3/1
  Integrator3/1 -> Create Diagonal Matrix/1, Sum7/2
  Create Diagonal Matrix/1 -> Matrix Multiply3/1
  Manual Switch1/1 -> M/1
  extract xy/1 -> Manual Switch1/1
  From20/1 -> Manual Switch1/2, extract xy/1
  extract xy1/1 -> Manual Switch2/1
  Manual Switch2/1 -> D/1
  From21/1 -> Manual Switch3/2, extract xy2/1
  extract xy2/1 -> Manual Switch3/1
  Manual Switch3/1 -> Sum2/3
  b_hat_body/1 -> Switch3/1
  Constant12/1 -> Matrix Multiply/1
  int_reset/1 -> Integrator1/2
  Constant10/1 -> Integrator1/3
  Ki/1 -> [Ki]
  Acc_est/1 -> Terminator/1
  Reshape/1 -> Matrix Multiply1/2
  "GNC: \"Transposed rotation matrix yaw: RTz_psi\"3"/1(R_T*eta_tilde) -> Goto16/1, Matrix Multiply4/1
  [Ki] -> Matrix Multiply4/2
  Matrix Multiply4/1 -> Switch3/3
  Int or bias comp/1 -> Switch3/2
  Int on/off/1 -> Switch2/2
  Switch3/1 -> Switch2/1
  Constant5/1 -> Switch2/3
  Switch2/1 -> tau_int/1
  tau/1 -> Terminator2/1, Goto13/1

== system ctrl_HSMBObserver/Hybrid Controller/Controllers/Tau ref. feedforward ==
  note: Model reference feewforward
      | term in Horisontal controller.
      | Martin Austad, 2003
  acc_des : Inport
  Nu_des : Inport  Port=2
  ref_scale : Inport  Port=3
  Enable : EnablePort
  Demux : Demux  Outputs=2
  Gain : Gain
  Gain1 : Gain  Gain=Control.PID.D  Multiplication=Matrix(K*u)  SaturateOnIntegerOverflow=on  OutDataTypeStr=Inherit: Same as input  ParamDataTypeStr=Inherit: Same as input
  Gain2 : Gain  Gain=Damping  Multiplication=Matrix(K*u)  SaturateOnIntegerOverflow=on  OutDataTypeStr=Inherit: Same as input  ParamDataTypeStr=Inherit: Same as input
  Gain3 : Gain  Gain=Control.PID.M  Multiplication=Matrix(K*u)  SaturateOnIntegerOverflow=on  OutDataTypeStr=Inherit: Same as input  ParamDataTypeStr=Inherit: Same as input
  Gain4 : Gain  Gain=Mass  Multiplication=Matrix(K*u)  SaturateOnIntegerOverflow=on  OutDataTypeStr=Inherit: Same as input  ParamDataTypeStr=Inherit: Same as input
  Manual Switch : ManualSwitch
  Manual Switch1 : ManualSwitch
  Product : Product
  Product1 : Product
  Sum : Sum  Inputs=+|+  SaturateOnIntegerOverflow=on
  tau_ff : Outport
  wires:
  Sum/1 -> Gain/1
  Nu_des/1 -> Gain1/1, Gain2/1
  Gain2/1 -> Manual Switch/2
  Gain1/1 -> Manual Switch/1
  Gain4/1 -> Manual Switch1/2
  Gain3/1 -> Manual Switch1/1
  acc_des/1 -> Gain4/1, Gain3/1
  Gain/1 -> tau_ff/1
  Manual Switch1/1 -> Product/1
  Product/1 -> Sum/2
  ref_scale/1 -> Demux/1
  Demux/1 -> [M_ref_scale]
  Demux/2 -> [D_ref_scale]
  Manual Switch/1 -> Product1/1
  Product1/1 -> Sum/1
  [D_ref_scale] -> Product1/2
  [M_ref_scale] -> Product/2

== system ctrl_HSMBObserver/Hybrid Controller/Fault Detection (freeze)/If Action Subsystem ==
  Action Port : ActionPort  ActionType=then
  Constant : Constant
  Constant1 : Constant  Value=diag([0 0 0])
  faultID : Outport
  pos_inject : Outport  Port=2
  wires:
  Constant/1 -> faultID/1
  Constant1/1 -> pos_inject/1

== system ctrl_HSMBObserver/Hybrid Controller/Fault Detection (freeze)/If Action Subsystem1 ==
  Action Port : ActionPort  ActionType=else
  Constant : Constant  Value=0
  Constant1 : Constant  Value=diag([1 1 1])
  faultID : Outport
  pos_inject : Outport  Port=2
  wires:
  Constant/1 -> faultID/1
  Constant1/1 -> pos_inject/1

== system ctrl_HSMBObserver/Hybrid Controller/Kinematic Observer Grip2015 + VVR1/Attitude Estimation1 ==
  lin acc meas : Inport
  compass meas : Inport  Port=2
  angular vel meas : Inport  Port=3
  hat f : Inport  Port=4
  Grip_reset : Inport  Port=5
  GripAttitude_gains2 : Inport  Port=6
  Constant1 : Constant  Value=eye(3)
  Constant2 : Constant  Value=[0;0;0]
  Gain : Gain
  Integrator1 : Integrator  ExternalReset=either  InitialConditionSource=external
  Integrator3 : Integrator  ExternalReset=either  InitialConditionSource=external
  Kp5 : Constant  Value=Obs.Grip2015.Mb
  Kp6 : Constant  Value=Obs.Grip2015.M_hatb
  MATLAB Function : MATLAB Function  Commented=on  TreatAsAtomicUnit=on
  MATLAB Function1 : MATLAB Function  TreatAsAtomicUnit=on
  MATLAB Function2 : MATLAB Function  TreatAsAtomicUnit=on
  MATLAB Function3 : MATLAB Function  TreatAsAtomicUnit=on
  MATLAB Function4 : MATLAB Function  TreatAsAtomicUnit=on
  Ma : Constant  Value=Obs.Grip2015.Ma
  Selector : Selector  InputPortWidth=7
  Selector1 : Selector  InputPortWidth=7  Indices=[2 3 4]
  Selector2 : Selector  InputPortWidth=7  Indices=[5 6 7]
  angular rate hat : Outport
  attitude hat : Outport  Port=2
  gyro bias hat : Outport  Port=3
  J hat : Outport  Port=4
  R hat : Outport  Port=5
  wires:
  MATLAB Function4/1(ang) -> attitude hat/1
  lin acc meas/1 -> MATLAB Function1/1(a_b)
  compass meas/1 -> MATLAB Function1/2(psi)
  [R_hat] -> MATLAB Function1/4(Rhat)
  Ma/1 -> MATLAB Function1/5(Ma)
  [Kp] -> MATLAB Function2/5(Kp)
  [Ki] -> MATLAB Function2/6(ki)
  Kp5/1 -> MATLAB Function2/3(Mb)
  Kp6/1 -> MATLAB Function2/4(Mbhat)
  MATLAB Function2/1(dot_bhat) -> Integrator1/1
  Integrator1/1 -> gyro bias hat/1, MATLAB Function2/7(bhat), Gain/1
  [R_hat] -> MATLAB Function3/2(Rhat)
  MATLAB Function3/2(rate_hat) -> angular rate hat/1
  MATLAB Function3/1(dot_Rhat) -> Integrator3/1
  angular vel meas/1 -> MATLAB Function3/3(Gyro_rate)
  MATLAB Function1/1(Jhat) -> MATLAB Function2/2(Jhat), MATLAB Function3/1(Jhat), J hat/1
  Integrator3/1 -> [R_hat], R hat/1
  [reset] -> Integrator1/2
  Constant2/1 -> Integrator1/3
  [reset] -> Integrator3/2
  Constant1/1 -> Integrator3/3
  Grip_reset/1 -> [reset]
  GripAttitude_gains2/1 -> Selector2/1, Selector1/1, Selector/1
  Selector/1 -> [sigma]
  Selector1/1 -> [Kp]
  Selector2/1 -> [Ki]
  [Kp] -> MATLAB Function3/6(Kp)
  [sigma] -> MATLAB Function3/5(Sigma)
  Gain/1 -> MATLAB Function3/4(bhat)
  hat f/1 -> MATLAB Function1/3(hatf_n)
  [R_hat] -> MATLAB Function2/1(Rhat)
  [R_hat] -> MATLAB Function4/1(R)

== system ctrl_HSMBObserver/Hybrid Controller/Kinematic Observer Grip2015 + VVR1/CG to MRU ==
  Pos CG : Inport
  Rotation matrix : Inport  Port=2
  Constant : Constant  Value=arm
  Matrix Multiply : Product  Multiplication=Matrix(*)
  Selector : Selector  InputPortWidth=3  Indices=[1 2]
  Sum : Sum  Inputs=|++
  Pos MRU : Outport
  wires:
  Pos CG/1 -> Sum/1
  Rotation matrix/1 -> Matrix Multiply/1
  Matrix Multiply/1 -> Selector/1
  Sum/1 -> Pos MRU/1
  Constant/1 -> Matrix Multiply/2
  Selector/1 -> Sum/2

== system ctrl_HSMBObserver/Hybrid Controller/Kinematic Observer Grip2015 + VVR1/Euler angles to inverse rotation matrix ==
  theta : Inport
  Mux2 : Mux  Inputs=2
  Mux3 : Mux  Inputs=9
  R11 : Fcn  Expr=u(5)*u(6)
  R12 : Fcn  Expr=u(5)*u(3)
  R13 : Fcn  Expr=-u(2)
  "R21 " : Fcn  Expr=-u(4)*u(3)+u(1)*u(2)*u(6)
  R22 : Fcn  Expr=u(4)*u(6)+u(1)*u(2)*u(3)
  R23 : Fcn  Expr=u(1)*u(5)
  "R31 " : Fcn  Expr=u(1)*u(3)+u(4)*u(2)*u(6)
  R32 : Fcn  Expr=-u(1)*u(6)+u(4)*u(2)*u(3)
  R33 : Fcn  Expr=u(4)*u(5)
  Reshape 9x1->3x3 : Reshape  OutputDimensionality=Customize  OutputDimensions=[3,3]
  cos(theta) : Trigonometry  Operator=cos
  sin(theta) : Trigonometry
  inv(R) : Outport  InitialOutput=0
  wires:
  Reshape 9x1->3x3/1 -> inv(R)/1
  R11/1 -> Mux3/1
  Mux3/1 -> Reshape 9x1->3x3/1
  sin(theta)/1 -> Mux2/1
  cos(theta)/1 -> Mux2/2
  theta/1 -> cos(theta)/1, sin(theta)/1
  Mux2/1 -> R32/1, R13/1, R33/1, R23/1, R22/1, "R31 "/1, R11/1, "R21 "/1, R12/1
  R23/1 -> Mux3/8
  R13/1 -> Mux3/7
  R22/1 -> Mux3/5
  R12/1 -> Mux3/4
  "R31 "/1 -> Mux3/3
  "R21 "/1 -> Mux3/2
  R32/1 -> Mux3/6
  R33/1 -> Mux3/9

== system ctrl_HSMBObserver/Hybrid Controller/Kinematic Observer Grip2015 + VVR1/Euler angles to inverse rotation matrix 2D ==
  theta : Inport
  Mux2 : Mux  Inputs=2
  Mux3 : Mux  Inputs=9
  R11 : Fcn  Expr=u(5)*u(6)
  R12 : Fcn  Expr=u(5)*u(3)
  R13 : Fcn  Expr=-u(2)
  "R21 " : Fcn  Expr=-u(4)*u(3)+u(1)*u(2)*u(6)
  R22 : Fcn  Expr=u(4)*u(6)+u(1)*u(2)*u(3)
  R23 : Fcn  Expr=u(1)*u(5)
  "R31 " : Fcn  Expr=u(1)*u(3)+u(4)*u(2)*u(6)
  R32 : Fcn  Expr=-u(1)*u(6)+u(4)*u(2)*u(3)
  R33 : Fcn  Expr=u(4)*u(5)
  Reshape 9x1->3x3 : Reshape  OutputDimensionality=Customize  OutputDimensions=[3,3]
  cos(theta) : Trigonometry  Operator=cos
  sin(theta) : Trigonometry
  inv(R) : Outport  InitialOutput=0
  wires:
  Reshape 9x1->3x3/1 -> inv(R)/1
  R11/1 -> Mux3/1
  Mux3/1 -> Reshape 9x1->3x3/1
  sin(theta)/1 -> Mux2/1
  cos(theta)/1 -> Mux2/2
  theta/1 -> cos(theta)/1, sin(theta)/1
  Mux2/1 -> R32/1, R13/1, R33/1, R23/1, R22/1, "R31 "/1, R11/1, "R21 "/1, R12/1
  R23/1 -> Mux3/8
  R13/1 -> Mux3/7
  R22/1 -> Mux3/5
  R12/1 -> Mux3/4
  "R31 "/1 -> Mux3/3
  "R21 "/1 -> Mux3/2
  R32/1 -> Mux3/6
  R33/1 -> Mux3/9

== system ctrl_HSMBObserver/Hybrid Controller/Kinematic Observer Grip2015 + VVR1/Linear position and velocity estimation1 ==
  note: Acc hat
  note: tilde pi
  note: hat pi
  note: z hat
  note: nu_hat
  note: pi
  note: tilde pi
  note: nu_hat
  note: nu_hat
  R hat : Inport
  hat J : Inport  Port=2
  Lin pos : Inport  Port=3
  acc_imu : Inport  Port=4
  Grip2015_gains : Inport  Port=5
  Grip_reset : Inport  Port=6
  Attitude gains : Inport  Port=7
  Constant2 : Constant  Value=[0;0;0]
  Constant3 : Constant  Value=[0;0;0]
  Constant4 : Constant  Value=[0;0;0]
  Constant5 : Constant  Value=0
  Integrator{1..4} (4 alike) : Integrator  ExternalReset=either  InitialConditionSource=external
  MATLAB Function1 : MATLAB Function  TreatAsAtomicUnit=on
  MATLAB Function2 : MATLAB Function  TreatAsAtomicUnit=on
  Matrix Multiply : Product  Multiplication=Matrix(*)
  Product6 : Product
  Selector : Selector  InputPortWidth=3  Indices=[3]
  Selector1 : Selector  InputPortWidth=10  Indices=10
  Selector3 : Selector  InputPortWidth=3  Indices=[1 2]
  Sum1 : Sum  Inputs=|++
  Sum2 : Sum  Inputs=++|
  Sum3 : Sum  Inputs=++|
  Sum4 : Sum  Inputs=+-
  Sum5 : Sum  Inputs=|++
  Sum6 : Sum  Inputs=-+|
  Sum7 : Sum  Inputs=++|
  Sum8 : Sum  Inputs=+-|
  VVR : Constant  Value=0
  gravity : Constant  Value=[0 0 Glob.g]
  force hat : Outport
  Lin pos hat : Outport  Port=2
  Lin vel hat : Outport  Port=3
  Lin acc hat : Outport  Port=4
  zeta : Outport  Port=5
  wires:
  Sum5/1 -> Integrator2/1
  Product6/1 -> Sum5/2
  Sum2/1 -> Integrator4/1
  Lin pos/1 -> Sum4/1
  Sum4/1 -> MATLAB Function2/2(e_pos)
  Integrator4/1 -> Selector/1, Selector3/1, Lin pos hat/1
  Selector3/1 -> Sum4/2
  VVR/1 -> Sum8/1
  Integrator2/1 -> Sum8/2
  R hat/1 -> Matrix Multiply/1
  acc_imu/1 -> MATLAB Function1/2(a_b), Matrix Multiply/2
  Matrix Multiply/1 -> Sum3/2
  Integrator1/1 -> zeta/1, Sum3/1
  Selector/1 -> Sum5/1
  Integrator3/1 -> Lin vel hat/1, Sum2/2
  Sum6/1 -> Integrator1/1
  hat J/1 -> MATLAB Function1/1(Jhat)
  Attitude gains/1 -> MATLAB Function1/3(AttGain)
  MATLAB Function1/1(y) -> Sum6/1
  Sum3/1 -> force hat/1, Sum1/1
  MATLAB Function2/1(corr_xi) -> Sum6/2
  MATLAB Function2/2(corr_v) -> Sum7/1
  MATLAB Function2/3(corr_p) -> Sum2/1
  Sum8/1 -> MATLAB Function2/3(e_vvr), Product6/1
  Grip_reset/1 -> [reset]
  Sum1/1 -> Lin acc hat/1, Sum7/2
  Sum7/1 -> Integrator3/1
  gravity/1 -> Sum1/2
  Grip2015_gains/1 -> [Gains]
  [Gains] -> MATLAB Function2/1(K)
  [Gains] -> Selector1/1
  Selector1/1 -> Product6/2
  [reset] -> Integrator3/2
  Constant2/1 -> Integrator3/3
  [reset] -> Integrator1/2
  Constant3/1 -> Integrator1/3
  [reset] -> Integrator4/2
  Constant4/1 -> Integrator4/3
  [reset] -> Integrator2/2
  Constant5/1 -> Integrator2/3

== system ctrl_HSMBObserver/Hybrid Controller/Kinematic Observer Grip2015 + VVR1/MRU to CG ==
  Rotation matrix : Inport
  Pos MRU : Inport  Port=2
  Constant : Constant  Value=arm
  Matrix Multiply : Product  Multiplication=Matrix(*)
  Selector : Selector  InputPortWidth=3  Indices=[1 2]
  Sum : Sum  Inputs=|+-
  Pos CG : Outport
  wires:
  Pos MRU/1 -> Sum/1
  Rotation matrix/1 -> Matrix Multiply/1
  Matrix Multiply/1 -> Selector/1
  Sum/1 -> Pos CG/1
  Constant/1 -> Matrix Multiply/2
  Selector/1 -> Sum/2

== system ctrl_HSMBObserver/Hybrid Controller/Nonlinear observer, version implemented 04.26.2016/Bias module ==
  note: Bias module
      | Uses bias time constant set in
      | "obsdat.m" when enabled. When
      | disabled --> Wiener process (T=0)
      | Martin Austad, 2003
  bias : Inport
  Enable : EnablePort
  T_inv : Gain  Gain=Control.VessObs.T_inv  Multiplication=Matrix(K*u)  SaturateOnIntegerOverflow=on  OutDataTypeStr=Inherit: Same as input  ParamDataTypeStr=Inherit: Same as input
  bias.dot : Outport
  wires:
  T_inv/1 -> bias.dot/1
  bias/1 -> T_inv/1
